simulink model "class_d_mfb"  (R2024b)
settings: Solver=VariableStepAuto  StartTime=0.0  StopTime=5e-3  MaxStep=1e-8  RelTol=1e-9
undefined symbols (not defined in the file): gaussian
libraries: simulink x2
settings Model: SimulationMode=rapid-accelerator  Creator=Aaron  LastModifiedBy=Aaron
settings SolverCC: ShapePreserveControl=EnableAll  ZeroCrossAlgorithm=Adaptive

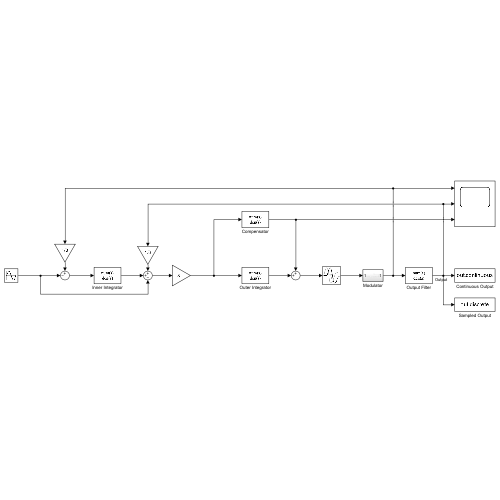
[thumbnail: Simulink's stored preview of the top-level diagram]
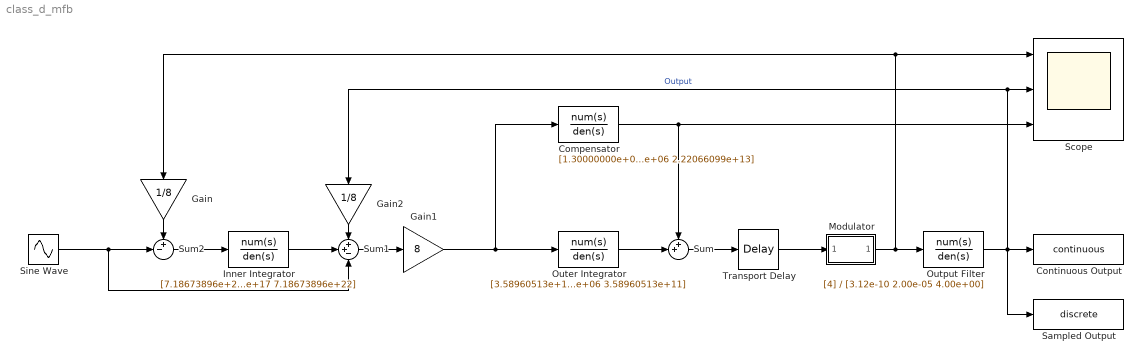
== system class_d_mfb ==
  Compensator : TransferFcn  Numerator=[1.30000000e+00 4.08407045e+06 3.20762143e+12]  Denominator=[1.00000000e+00 9.42477796e+06 2.22066099e+13]
  Continuous Output : ToWorkspace  VariableName=continuous  SaveFormat=Structure With Time  SampleTime=-1
  Gain : Gain  Gain=1/8
  Gain1 : Gain  Gain=8
  Gain2 : Gain  Gain=1/8
  Inner Integrator : TransferFcn  Numerator=[7.18673896e+22]  Denominator=[1.00000000e+00 3.05817794e+06 2.87153768e+12 8.22569044e+17 7.18673896e+22]
  Modulator : Subsystem
  Outer Integrator : TransferFcn  Numerator=[3.58960513e+11]  Denominator=[1.00000000e+00 1.11648114e+06 3.58960513e+11]
  Output Filter : TransferFcn  Numerator=[4]  Denominator=[3.12e-10 2.00e-05 4.00e+00]
  Sampled Output : ToWorkspace  VariableName=discrete  SampleTime=-1
  Scope : Scope  NumInputPorts=3
  Sine Wave : Sin  Amplitude=4  Frequency=2*pi*1e3  SampleTime=0
  Sum : Sum  Inputs=++|
  Sum1 : Sum  Inputs=++-
  Sum2 : Sum  Inputs=+-|
  Transport Delay : TransportDelay  DelayTime=60e-9
  wires:
  Transport Delay/1 -> Modulator/1(Input)
  Modulator/1(Output) -> Scope/1, Gain/1, Output Filter/1
  Sum/1 -> Transport Delay/1
  Outer Integrator/1 -> Sum/2
  Compensator/1 -> Scope/3, Sum/1
  Output Filter/1 -> Sampled Output/1, Continuous Output/1, Scope/2, Gain2/1  "Output"
  Sum1/1 -> Gain1/1
  Sine Wave/1 -> Sum2/2, Sum1/3
  Inner Integrator/1 -> Sum1/2
  Gain/1 -> Sum2/1
  Sum2/1 -> Inner Integrator/1
  Gain1/1 -> Compensator/1, Outer Integrator/1
  Gain2/1 -> Sum1/1

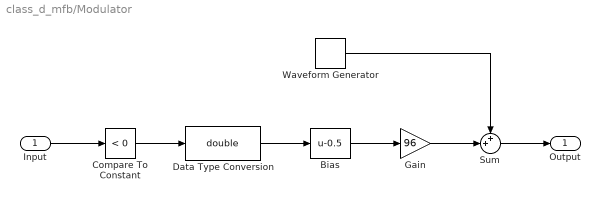
== system class_d_mfb/Modulator ==
  Input : Inport
  Bias : Bias  Bias=-0.5  SaturateOnIntegerOverflow=off
  Compare To Constant : simulink/Logic and Bit Operations/Compare To Constant  relop=<  const=0  OutDataTypeStr=uint8
  Data Type Conversion : DataTypeConversion  OutDataTypeStr=double  SaturateOnIntegerOverflow=off  RndMeth=Floor
  Gain : Gain  Gain=96
  Sum : Sum  Inputs=++|
  Waveform Generator : simulink/Sources/Waveform Generator  OutMin=[]  OutMax=[]  OutDataTypeStr=double  SelectedSignal=1  Signals=gaussian('Variance',1e-1)  BlockNames=MultiportSwitch_21ebdc26c22b472  SampleTime=0.1
  Output : Outport
  wires:
  Input/1 -> Compare To Constant/1
  Data Type Conversion/1 -> Bias/1
  Compare To Constant/1 -> Data Type Conversion/1
  Bias/1 -> Gain/1
  Waveform Generator/1 -> Sum/1
  Gain/1 -> Sum/2
  Sum/1 -> Output/1
